simulink model "PP_model"  (R2022b)
settings: Solver=VariableStepAuto  StartTime=0.0  StopTime=10.0  RelTol=1e-3
settings Model: Creator=tilog  LastModifiedBy=tilog

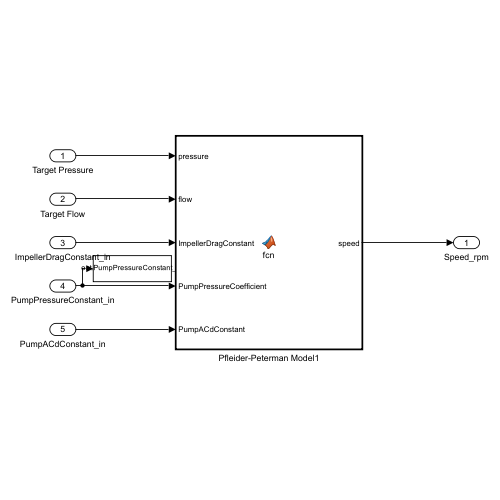
[thumbnail: Simulink's stored preview of the top-level diagram]
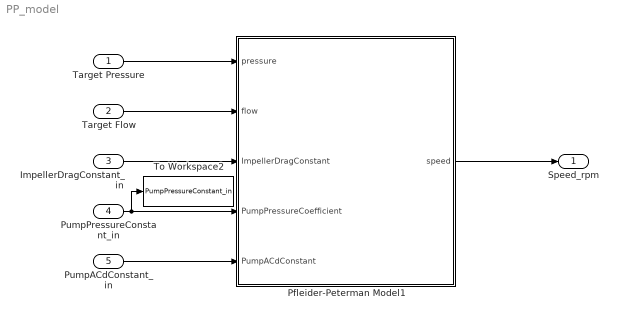
== system PP_model ==
  Target Pressure : Inport
  Target Flow : Inport  Port=2
  ImpellerDragConstant_in : Inport  Port=3
  PumpPressureConstant_in : Inport  Port=4
  PumpACdConstant_in : Inport  Port=5
  Pfleider-Peterman Model1 : MATLAB Function  TreatAsAtomicUnit=on
  To Workspace2 : ToWorkspace  VariableName=PumpPressureConstant_in  SaveFormat=Structure With Time  SampleTime=-1
  Speed_rpm : Outport
  wires:
  Target Flow/1 -> Pfleider-Peterman Model1/2(flow)
  Target Pressure/1 -> Pfleider-Peterman Model1/1(pressure)
  Pfleider-Peterman Model1/1(speed) -> Speed_rpm/1
  ImpellerDragConstant_in/1 -> Pfleider-Peterman Model1/3(ImpellerDragConstant)
  PumpACdConstant_in/1 -> Pfleider-Peterman Model1/5(PumpACdConstant)
  PumpPressureConstant_in/1 -> To Workspace2/1, Pfleider-Peterman Model1/4(PumpPressureCoefficient)

== matlab function PP_model/Pfleider-Peterman Model1 ==
  data: pressure input; flow input; speed output; ImpellerDragConstant input; PumpPressureCoefficient input; PumpACdConstant input
function speed = fcn( ...
    pressure, ...
    flow, ...
    ImpellerDragConstant, ...
    PumpPressureCoefficient, ... ...
    PumpACdConstant ...
    )

a = PumpPressureCoefficient;
b = -1 * ImpellerDragConstant * flow;
c = (-1*pressure) - ((flow^2)/PumpACdConstant);
speed = (-b + sqrt((b^2)-(4*a*c)))/(2*a);
